simulink model "Peak_Shave_Model"  (R2020a)
settings: Solver=VariableStepAuto  StartTime=0.0  StopTime=23  FixedStep=0.001  RelTol=1e-3
undefined symbols (not defined in the file): auxPower, BESSCapacity, chargeSetting, dischargeSetting, efficiency, ratedPower, ratedPowerNEG
libraries: simulink x8
settings Model: Creator=jeffm  LastModifiedBy=jeffm
settings DataIOCC: ExternalInput=ts  LoadExternalInput=on

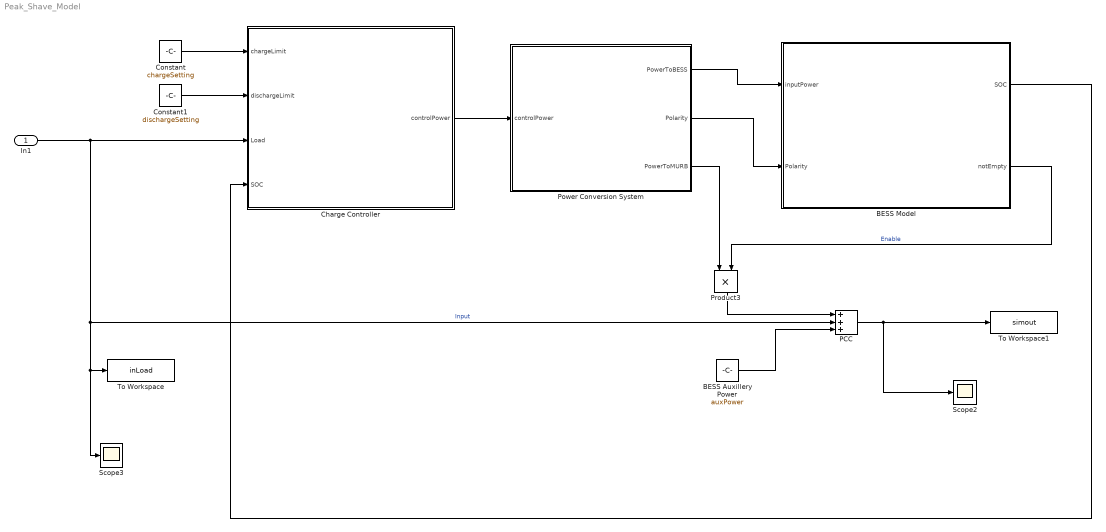
== system Peak_Shave_Model ==
  In1 : Inport
  BESS Auxillery Power : Constant  Value=auxPower  VectorParams1D=off
  BESS Model : Subsystem
  Charge Controller : Subsystem
  Constant : Constant  Value=chargeSetting
      settings: AttributesFormatString=%<Value>
  Constant1 : Constant  Value=dischargeSetting
      settings: AttributesFormatString=%<Value>
  PCC : Sum  Inputs=+++
  Power Conversion System : Subsystem
  Product3 : Product
  Scope2 : Scope
  Scope3 : Scope
  To Workspace : ToWorkspace  VariableName=inLoad  SaveFormat=Timeseries  SampleTime=-1
  To Workspace1 : ToWorkspace  VariableName=simout  SaveFormat=Timeseries  SampleTime=-1
  wires:
  In1/1 -> To Workspace/1, Scope3/1, PCC/2, Charge Controller/3(Load)  "Input"
  Product3/1 -> PCC/1
  BESS Auxillery Power/1 -> PCC/3
  PCC/1 -> Scope2/1, To Workspace1/1
  Constant/1 -> Charge Controller/1(chargeLimit)
  Constant1/1 -> Charge Controller/2(dischargeLimit)
  Charge Controller/1(controlPower) -> Power Conversion System/1(controlPower)
  Power Conversion System/3(PowerToMURB) -> Product3/1
  Power Conversion System/1(PowerToBESS) -> BESS Model/1(inputPower)
  BESS Model/1(SOC) -> Charge Controller/4(SOC)
  BESS Model/2(notEmpty) -> Product3/2  "Enable"
  Power Conversion System/2(Polarity) -> BESS Model/2(Polarity)

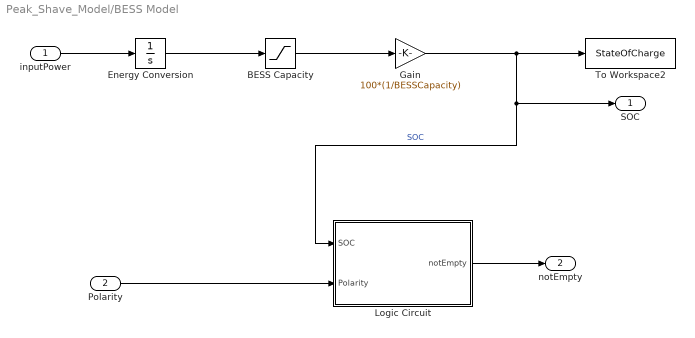
== system Peak_Shave_Model/BESS Model ==
  inputPower : Inport
  Polarity : Inport  Port=2
  BESS Capacity : Saturate  UpperLimit=BESSCapacity  LowerLimit=0
  Energy Conversion : Integrator
  Gain : Gain  Gain=100*(1/BESSCapacity)
  Logic Circuit : Subsystem
  To Workspace2 : ToWorkspace  VariableName=StateOfCharge  SaveFormat=Timeseries  SampleTime=-1
  SOC : Outport
  notEmpty : Outport  Port=2
  wires:
  Energy Conversion/1 -> BESS Capacity/1
  BESS Capacity/1 -> Gain/1
  Gain/1 -> To Workspace2/1, Logic Circuit/1(SOC), SOC/1  "SOC"
  inputPower/1 -> Energy Conversion/1
  Polarity/1 -> Logic Circuit/2(Polarity)
  Logic Circuit/1(notEmpty) -> notEmpty/1

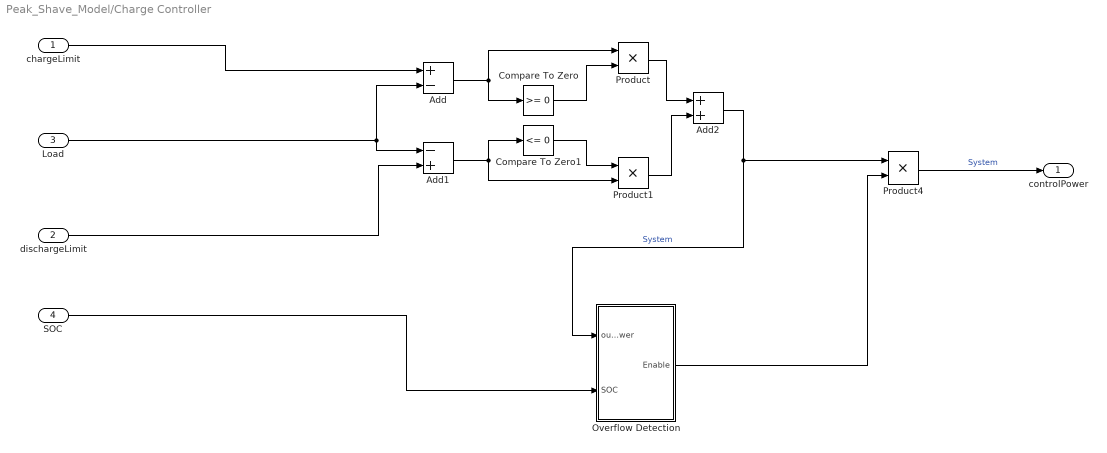
== system Peak_Shave_Model/Charge Controller ==
  chargeLimit : Inport
  dischargeLimit : Inport  Port=2
  Load : Inport  Port=3
  SOC : Inport  Port=4
  Add : Sum  Inputs=+-
  Add1 : Sum  Inputs=-+
  Add2 : Sum
  Compare To Zero : simulink/Logic and Bit Operations/Compare To Zero  relop=>=  OutDataTypeStr=boolean
  Compare To Zero1 : simulink/Logic and Bit Operations/Compare To Zero  relop=<=  OutDataTypeStr=boolean
  Overflow Detection : Subsystem
  Product : Product
  Product1 : Product
  Product4 : Product
  controlPower : Outport
  wires:
  Compare To Zero/1 -> Product/2
  Add/1 -> Compare To Zero/1, Product/1
  Overflow Detection/1(Enable) -> Product4/2
  Add1/1 -> Compare To Zero1/1, Product1/2
  Compare To Zero1/1 -> Product1/1
  Product/1 -> Add2/1
  Load/1 -> Add1/1, Add/2
  Add2/1 -> Overflow Detection/1(outputPower), Product4/1  "System"
  Product1/1 -> Add2/2
  SOC/1 -> Overflow Detection/2(SOC)
  chargeLimit/1 -> Add/1
  Product4/1 -> controlPower/1  "System"
  dischargeLimit/1 -> Add1/2

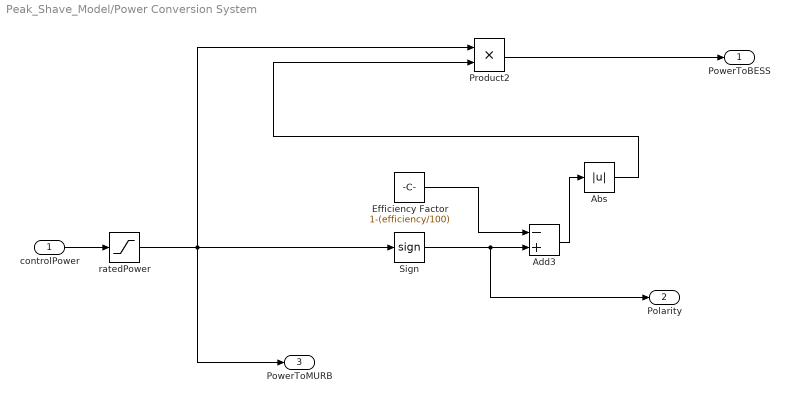
== system Peak_Shave_Model/Power Conversion System ==
  controlPower : Inport
  Abs : Abs
  Add3 : Sum  Inputs=-+
  Efficiency Factor : Constant  Value=1-(efficiency/100)
  Product2 : Product
  Sign : Signum
  ratedPower : Saturate  UpperLimit=ratedPower  LowerLimit=ratedPowerNEG
  PowerToBESS : Outport
  Polarity : Outport  Port=2
  PowerToMURB : Outport  Port=3
  wires:
  ratedPower/1 -> PowerToMURB/1, Sign/1, Product2/1
  Abs/1 -> Product2/2
  controlPower/1 -> ratedPower/1
  Sign/1 -> Add3/2, Polarity/1
  Add3/1 -> Abs/1
  Product2/1 -> PowerToBESS/1
  Efficiency Factor/1 -> Add3/1

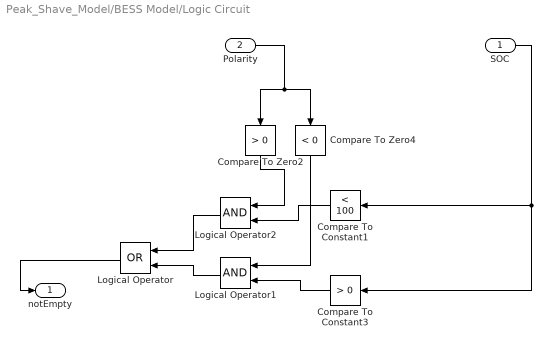
== system Peak_Shave_Model/BESS Model/Logic Circuit ==
  SOC : Inport
  Polarity : Inport  Port=2
  Compare To Constant1 : simulink/Logic and Bit Operations/Compare To Constant  relop=<  const=100  OutDataTypeStr=boolean
  Compare To Constant3 : simulink/Logic and Bit Operations/Compare To Constant  relop=>  const=0  OutDataTypeStr=boolean
  Compare To Zero2 : simulink/Logic and Bit Operations/Compare To Zero  relop=>  OutDataTypeStr=boolean
  Compare To Zero4 : simulink/Logic and Bit Operations/Compare To Zero  relop=<  OutDataTypeStr=boolean
  Logical Operator : Logic  Operator=OR  AllPortsSameDT=off  OutDataTypeStr=boolean
  Logical Operator1 : Logic  AllPortsSameDT=off  OutDataTypeStr=boolean
  Logical Operator2 : Logic  AllPortsSameDT=off  OutDataTypeStr=boolean
  notEmpty : Outport
  wires:
  SOC/1 -> Compare To Constant3/1, Compare To Constant1/1
  Logical Operator1/1 -> Logical Operator/2
  Compare To Zero4/1 -> Logical Operator1/1
  Compare To Zero2/1 -> Logical Operator2/1
  Logical Operator2/1 -> Logical Operator/1
  Polarity/1 -> Compare To Zero2/1, Compare To Zero4/1
  Logical Operator/1 -> notEmpty/1
  Compare To Constant3/1 -> Logical Operator1/2
  Compare To Constant1/1 -> Logical Operator2/2

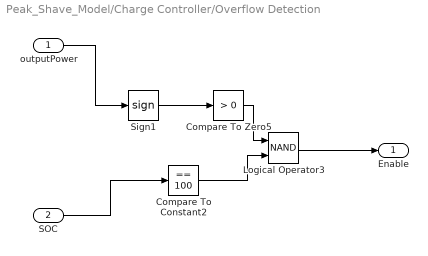
== system Peak_Shave_Model/Charge Controller/Overflow Detection ==
  outputPower : Inport
  SOC : Inport  Port=2
  Compare To Constant2 : simulink/Logic and Bit Operations/Compare To Constant  relop===  const=100  OutDataTypeStr=boolean
  Compare To Zero5 : simulink/Logic and Bit Operations/Compare To Zero  relop=>  OutDataTypeStr=boolean
  Logical Operator3 : Logic  Operator=NAND  AllPortsSameDT=off  OutDataTypeStr=boolean
  Sign1 : Signum
  Enable : Outport
  wires:
  Compare To Constant2/1 -> Logical Operator3/2
  Compare To Zero5/1 -> Logical Operator3/1
  Sign1/1 -> Compare To Zero5/1
  Logical Operator3/1 -> Enable/1
  outputPower/1 -> Sign1/1
  SOC/1 -> Compare To Constant2/1
